simulink model "Final_Project"  (R2020b)
settings: Solver=VariableStepAuto  StartTime=0.0  StopTime=10.0  MaxStep=0.5e-5  RelTol=1e-3
libraries: nesl_utility x11, ee_lib x10, fl_lib x9, simulink x2
settings Model: Creator=edoardo  LastModifiedBy=edoardo
settings SolverCC: ZeroCrossAlgorithm=Adaptive
settings DebuggingCC: IgnoredZcDiagnostic=none

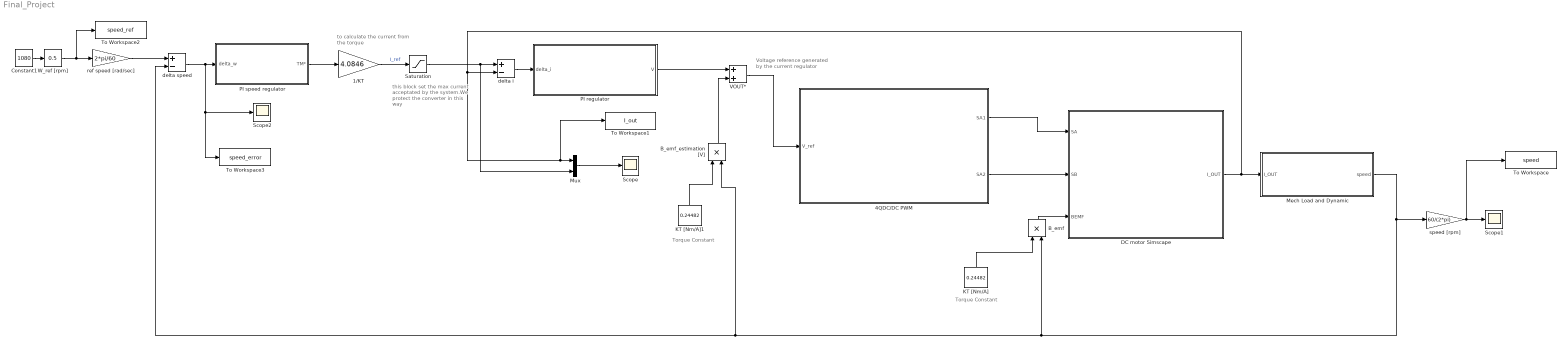
== system Final_Project ==
  note: Voltage reference generated
      | by the current regulator
  note: Torque Constant
  note: to calculate the current
      | from the torque
  note: this block set the max
      | current acceptated by the
      | system.We protect the
      | converter in this way
  note: Torque Constant
  " B_emf " : Product
  " B_emf_estimation [V]" : Product
  1/KT : Gain  Gain=4.0846
  4QDC/DC PWM : Subsystem
  Constant1 : Constant  Value=1080
  DC motor Simscape : Subsystem
  KT [Nm/A] : Constant  Value=0.24482
  KT [Nm/A]1 : Constant  Value=0.24482
  Mech Load and Dynamic : Subsystem
  Mux : Mux  Inputs=2
  PI regulator : Subsystem
  PI speed regulator : Subsystem
  Saturation : Saturate  UpperLimit=1.4  LowerLimit=-1.4
  Scope : Scope
  Scope1 : Scope
  Scope2 : Scope
  To Workspace : ToWorkspace  VariableName=speed  SaveFormat=Timeseries  SampleTime=-1
  To Workspace1 : ToWorkspace  VariableName=I_out  SaveFormat=Timeseries  SampleTime=-1
  To Workspace2 : ToWorkspace  VariableName=speed_ref  SaveFormat=Timeseries  SampleTime=-1
  To Workspace3 : ToWorkspace  VariableName=speed_error  SaveFormat=Timeseries  SampleTime=-1
  VOUT* : Sum
  W_ref [rpm] : simulink/Math Operations/Slider Gain  gain=0.5  low=-1  high=1
  "delta i " : Sum  Inputs=+-
  delta speed : Sum  Inputs=+-
  "ref speed [rad/sec] " : Gain  Gain=2*pi/60
  speed [rpm] : Gain  Gain=60/(2*pi)
  wires:
  KT [Nm/A]1/1 -> " B_emf_estimation [V]"/1
  " B_emf_estimation [V]"/1 -> VOUT*/2
  W_ref [rpm]/1 -> To Workspace2/1, "ref speed [rad/sec] "/1
  Constant1/1 -> W_ref [rpm]/1
  delta speed/1 -> Scope2/1, To Workspace3/1, PI speed regulator/1(delta_w)
  1/KT/1 -> Saturation/1  "I_ref"
  speed [rpm]/1 -> To Workspace/1, Scope1/1
  Saturation/1 -> Mux/2, "delta i "/1
  "ref speed [rad/sec] "/1 -> delta speed/1
  Mux/1 -> Scope/1
  DC motor Simscape/1(I_OUT) -> Mech Load and Dynamic/1(I_OUT), "delta i "/2, To Workspace1/1, Mux/1
  VOUT*/1 -> 4QDC/DC PWM/1(V_ref)
  "delta i "/1 -> PI regulator/1(delta_i)
  PI regulator/1(V) -> VOUT*/1
  PI speed regulator/1(TM*) -> 1/KT/1
  4QDC/DC PWM/1(SA1) -> DC motor Simscape/1(SA)
  4QDC/DC PWM/2(SA2) -> DC motor Simscape/2(SB)
  KT [Nm/A]/1 -> " B_emf "/1
  " B_emf "/1 -> DC motor Simscape/3(BEMF)
  Mech Load and Dynamic/1(speed) -> speed [rpm]/1, " B_emf "/2, " B_emf_estimation [V]"/2, delta speed/2

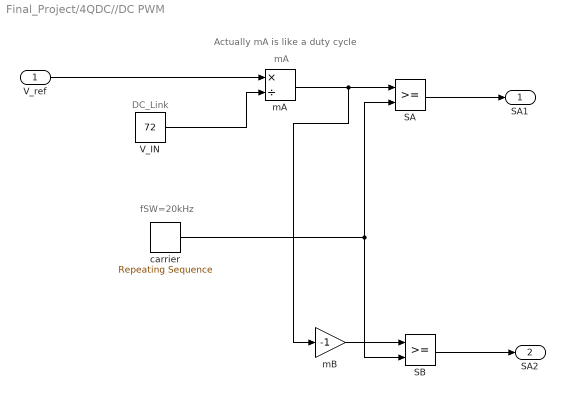
== system Final_Project/4QDC//DC PWM ==
  note: Actually mA is like a duty cycle
  note: DC_Link
  note: fSW=20kHz
  note: mA
  V_ref : Inport
  SA : RelationalOperator  OutDataTypeStr=boolean  RndMeth=Simplest
  SB : RelationalOperator  OutDataTypeStr=boolean  RndMeth=Simplest
  V_IN : Constant  Value=72
  carrier : simulink/Sources/Repeating Sequence  rep_seq_t=[0 0.5e-4/2 0.5e-4]  rep_seq_y=[-1 1 -1]
  mA : Product  Inputs=*/
  mB : Gain  Gain=-1
  SA1 : Outport
  SA2 : Outport  Port=2
  wires:
  V_ref/1 -> mA/1
  carrier/1 -> SA/2, SB/2
  mA/1 -> mB/1, SA/1
  SB/1 -> SA2/1
  mB/1 -> SB/1
  V_IN/1 -> mA/2
  SA/1 -> SA1/1

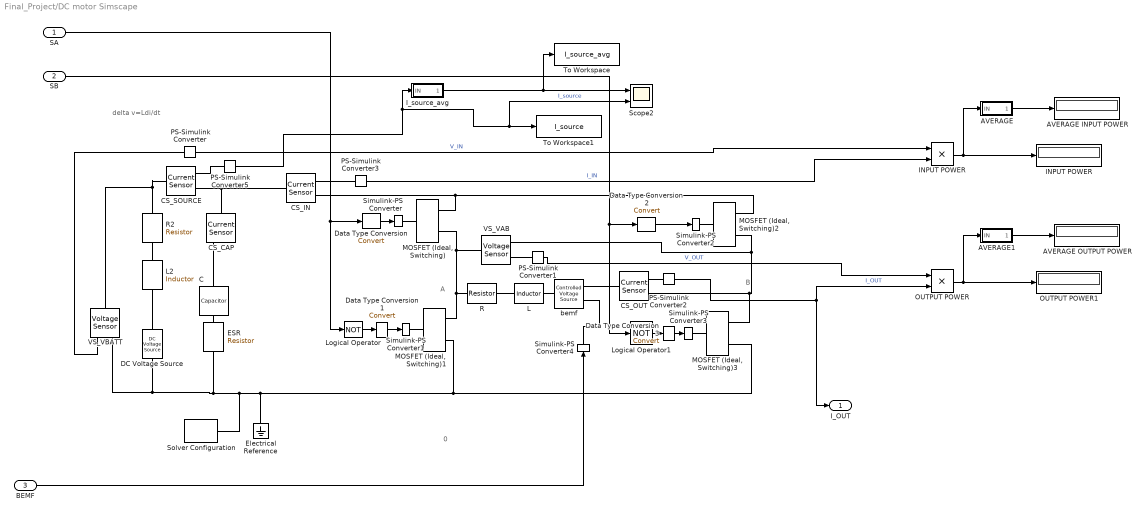
== system Final_Project/DC motor Simscape ==
  note: delta v=Ldi/dt
  note: B
  note: 0
  note: A
  SA : Inport
  SB : Inport  Port=2
  BEMF : Inport  Port=3
  " INPUT POWER" : Display
  AVERAGE : Subsystem  mask{Ts=0.0001}
      mask prompts: Ts "period"
  AVERAGE INPUT POWER : Display
  AVERAGE OUTPUT POWER : Display
  AVERAGE1 : Subsystem  mask{Ts=0.0001}
      mask prompts: Ts "period"
  C : ee_lib/Passive/Capacitor  cap_option=0  c=1e-4 F  Cvec=[1e-05, 1e-06] F  Vvec=[0, 10] V  CV_table_symmetry=1  f_vec=[1, 10] kHz  DFext_vec=[.8, 1.2]  C_tol=5  enable_C_tol=0  tol_distribution=1  nSigma=4  r=1e-6 Ohm  g=0 1/Ohm  averaging_period=0 s  enable_operating_limits=0  operating_limit_action=2  max_working_voltage_range=[-25, 25] V  power_rating=1 W  enable_faults=0  fault_action=1  Cscale_faulted=100  R_faulted=1e-3 Ohm  G_faulted=0 1/Ohm  tau_fault=1e-3 s  enable_temporal_fault=0  t_fault=1 s  enable_behavioral_fault=0  max_permissible_voltage_range=[-100, 100] V  t_fail_on_voltage=1 s  i_specify=off  i_priority=None  i=0 A  i_nominal_specify=off  i_nominal_unit=A  i_nominal_value=1  v_specify=off  v_priority=None  v=0 V  v_nominal_specify=off  v_nominal_unit=V  v_nominal_value=1  vc_specify=off  vc_priority=High  vc=0 V  vc_nominal_specify=off  vc_nominal_unit=V  vc_nominal_value=1
  CS_CAP : fl_lib/Electrical/Electrical Sensors/Current Sensor
  CS_IN : fl_lib/Electrical/Electrical Sensors/Current Sensor
  CS_OUT : fl_lib/Electrical/Electrical Sensors/Current Sensor
  CS_SOURCE : fl_lib/Electrical/Electrical Sensors/Current Sensor
  DC Voltage Source : fl_lib/Electrical/Electrical Sources/DC Voltage Source  v0=72 V
  Data Type Conversion{,1..3} (4 alike) : DataTypeConversion
  ESR : ee_lib/Passive/Resistor  R=0.01 Ohm  R_tol=5  enable_R_tol=0  tol_distribution=1  nSigma=4  enable_operating_limits=0  operating_limit_action=2  max_working_voltage=100 V  power_rating=1 W  enable_faults=0  fault_action=1  R_faulted=inf Ohm  enable_temporal_fault=0  t_fault=1 s  enable_behavioral_fault=0  max_permissible_current=1 A  t_fail_on_current=1 s  noise_mode=0  sample_time=1e-3 s  repeatability=1  auto_seed=3922919431  user_seed=0  Tdevice=25 degC  alpha=3.93e-3 1/K  Tmeas=25 degC  thermal_mass=100 J/K  power_derating_T1=70 degC  power_derating_T2=155 degC  operating_temperature_range_vec=[-50, 150] degC  temperature_specify=off  temperature_priority=High  temperature=298.15 K  temperature_nominal_specify=off  temperature_nominal_unit=K  temperature_nominal_value=1
  Electrical Reference : fl_lib/Electrical/Electrical Elements/Electrical Reference
  INPUT POWER : Product
  I_source_avg : Subsystem  mask{Ts=0.0001}
      mask prompts: Ts "period"
  L : ee_lib/Passive/Inductor  l=6.4e-3 H  L_tol=20  enable_L_tol=0  tol_distribution=1  nSigma=4  r=0 Ohm  g=1e-9 1/Ohm  enable_operating_limits=0  operating_limit_action=2  max_working_current=1 A  power_rating=1 W  enable_faults=0  fault_action=1  lambdaPercent=50  k_faulted=0.9999  turnsShort=0  openCct=0  groundShort=0  groundShortG=0 1/Ohm  tau_fault=1e-3 s  enable_temporal_fault=0  t_fault=1 s  enable_behavioral_fault=0  max_permissible_voltage=100 V  n_fail_on_voltage=1  max_permissible_current=1 A  t_fail_on_current=1 s  i_L_specify=off  i_L_priority=High  i_L=0 A  i_L_nominal_specify=off  i_L_nominal_unit=A  i_L_nominal_value=1
  L2 : ee_lib/Passive/Inductor  l=0.72e-3 H  L_tol=20  enable_L_tol=0  tol_distribution=1  nSigma=4  r=0 Ohm  g=1e-9 1/Ohm  enable_operating_limits=0  operating_limit_action=2  max_working_current=1 A  power_rating=1 W  enable_faults=0  fault_action=1  lambdaPercent=50  k_faulted=0.9999  turnsShort=0  openCct=0  groundShort=0  groundShortG=0 1/Ohm  tau_fault=1e-3 s  enable_temporal_fault=0  t_fault=1 s  enable_behavioral_fault=0  max_permissible_voltage=100 V  n_fail_on_voltage=1  max_permissible_current=1 A  t_fail_on_current=1 s  i_L_specify=off  i_L_priority=High  i_L=0 A  i_L_nominal_specify=off  i_L_nominal_unit=A  i_L_nominal_value=1
  Logical Operator : Logic  Operator=NOT  AllPortsSameDT=off  OutDataTypeStr=boolean
  Logical Operator1 : Logic  Operator=NOT  AllPortsSameDT=off  OutDataTypeStr=boolean
  MOSFET (Ideal, Switching){,1..3} (4 alike) : ee_lib/Semiconductors & Converters/MOSFET (Ideal, Switching)  Rds=0.1 Ohm  Goff=1e-6 1/Ohm  Vth=0.5 V  diode_param=1  diode_Vf=0.8 V  diode_Ron=0.001 Ohm  diode_Goff=1e-5 1/Ohm  diode_C=50e-9 F  diode_iRM=-235 A  diode_iF=300 A  diode_idot=-50 A/us  diode_trr_param=1  diode_trr_factor=3  diode_trr=15 us  diode_Qrr=1500 s*uA  thermal_loss_option=2  Von_data=[0, 1.1, 1.3, 1.45, 1.75, 2.25, 2.7; 0, 1, 1.15, 1.35, 1.7, 2.35, 3] V  Eon_data=[0, .29, 1.43, 2.86, 5.71, 13.14, 22.86; 0, .57, 2.63, 5.14, 10.29, 20.57, 30.29] * 1e-3 J  Eoff_data=[0, .21, 1.07, 2.14, 4.29, 9.86, 17.14; 0, .43, 1.97, 3.86, 7.71, 15.43, 22.71] * 1e-3 J  Tj=[298.15, 398.15] K  Iout_data=[0, 10, 50, 100, 200, 400, 600] A  Eon_scalar=22.86e-3 J  Eoff_scalar=17.14e-3 J  Voff=300 V  Iout_scalar=600 A  diodeModelType=ee.enum.converters.diodeModelType.pwl  diode_IfMat=[.07, .12, .19, 1.75, 4.24, 7.32, 11.2; .16, .3, .72, 2.14, 4.02, 6.35, 9.12] A  diode_TjVec=[25, 125] degC  diode_VfVec=[.5, .7, .9, 1.3, 1.7, 2.1, 2.5] V  thermal_network_parameterization=ee.enum.thermalNetworkTopology.external  Rth=[.03, .2] K/W  Rth_Foster=[.03, .2] K/W  thermal_mass_parameterization=ee.enum.thermalNetwork.timeconstant  thermal_mass=[3, 25] J/K  thermal_mass_Foster=[33, 50] J/K  thermal_time_constant=[.1, 5] s  thermal_time_constant_Foster=[1, 10] s  thermal_mass_initial_temperatures=[25, 25] degC  junction_thermal_mass=0.1 J/K  Tau=1e-4 s  vT_specify=off  vT_priority=None  vT=0 V  vT_nominal_specify=off  vT_nominal_unit=V  vT_nominal_value=1  Qj_specify=off  Qj_priority=None  Qj=0 W  Qj_nominal_specify=off  Qj_nominal_unit=W  Qj_nominal_value=1  junction_temperature_specify=off  junction_temperature_priority=None  junction_temperature=25 degC  junction_temperature_nominal_specify=off  junction_temperature_nominal_unit=degC  junction_temperature_nominal_value=1
  OUTPUT POWER : Product
  OUTPUT POWER1 : Display
  PS-Simulink Converter{,1..3,5} (5 alike) : nesl_utility/PS-Simulink Converter  PhysicalDomain=network_engine_domain  SubClassName=ps_output  LeftPortType=input  RightPortType=output  PseudoPeriodic=off  Frequencies=[]  Unit=1  AffineConversion=off
  R : ee_lib/Passive/Resistor  R=24.9 Ohm  R_tol=5  enable_R_tol=0  tol_distribution=1  nSigma=4  enable_operating_limits=0  operating_limit_action=2  max_working_voltage=100 V  power_rating=1 W  enable_faults=0  fault_action=1  R_faulted=inf Ohm  enable_temporal_fault=0  t_fault=1 s  enable_behavioral_fault=0  max_permissible_current=1 A  t_fail_on_current=1 s  noise_mode=0  sample_time=1e-3 s  repeatability=1  auto_seed=2715962282  user_seed=0  Tdevice=25 degC  alpha=3.93e-3 1/K  Tmeas=25 degC  thermal_mass=100 J/K  power_derating_T1=70 degC  power_derating_T2=155 degC  operating_temperature_range_vec=[-50, 150] degC  temperature_specify=off  temperature_priority=High  temperature=298.15 K  temperature_nominal_specify=off  temperature_nominal_unit=K  temperature_nominal_value=1
  R2 : ee_lib/Passive/Resistor  R=0.3 Ohm  R_tol=5  enable_R_tol=0  tol_distribution=1  nSigma=4  enable_operating_limits=0  operating_limit_action=2  max_working_voltage=100 V  power_rating=1 W  enable_faults=0  fault_action=1  R_faulted=inf Ohm  enable_temporal_fault=0  t_fault=1 s  enable_behavioral_fault=0  max_permissible_current=1 A  t_fail_on_current=1 s  noise_mode=0  sample_time=1e-3 s  repeatability=1  auto_seed=418932850  user_seed=0  Tdevice=25 degC  alpha=3.93e-3 1/K  Tmeas=25 degC  thermal_mass=100 J/K  power_derating_T1=70 degC  power_derating_T2=155 degC  operating_temperature_range_vec=[-50, 150] degC  temperature_specify=off  temperature_priority=High  temperature=298.15 K  temperature_nominal_specify=off  temperature_nominal_unit=K  temperature_nominal_value=1
  Scope2 : Scope  NumInputPorts=2
  Simulink-PS Converter{,1..4} (5 alike) : nesl_utility/Simulink-PS Converter  PhysicalDomain=network_engine_domain  SubClassName=ps_input  LeftPortType=input  RightPortType=output  PseudoPeriodic=off  Frequencies=[]  NoiseDistribution=none  NoiseParameters=[]  Unit=1  AffineConversion=off  FilteringAndDerivatives=provide  SimscapeFilterOrder=1  InputFilterTimeConstant=0.001  UdotUserProvided=0
  Solver Configuration : nesl_utility/Solver Configuration  PhysicalDomain=network_engine_domain  SubClassName=solver  LeftPortType=input  RightPortType=generic  Tones=[]  Harmonics=[]  SimulateNoise=off  Profile=off  UseLocalSampling=off  EnableSwitchedLinearOptims=on  FrequencyDomain=off  UseCCode=off  RelTol=0.001  AbsTol=1e-06  MinStep=1e-09  ToWorkspace=off  RevertToSquareIcSolve=off  NumHomotopyIterations=100  PhasorMode=off  PhasorModeNumHarmonics=1  DoDC=off  ResidualTolerance=1e-09  UseLocalSolver=off  LocalSolverChoice=NE_BACKWARD_EULER_ADVANCER  LocalSolverSampleTime=0.001  DoFixedCost=off  MaxNonlinIter=3  MaxModeIter=2  ComputeImpulses=off  ImpulseIterations=2  LinearAlgebra=auto  EquationFormulation=NE_TIME_EF  DelaysMemoryBudget=1024  AutomaticFiltering=on  FilteringTimeConstant=0.001  PartitionStorageMethod=AS_NEEDED  PartitionMemoryBudget=1024  PartitionMethod=ROBUST
  To Workspace : ToWorkspace  VariableName=I_source_avg  SaveFormat=Timeseries  SampleTime=-1
  To Workspace1 : ToWorkspace  VariableName=I_source  SaveFormat=Timeseries  SampleTime=-1
  VS_VAB : fl_lib/Electrical/Electrical Sensors/Voltage Sensor
  VS_VBATT : fl_lib/Electrical/Electrical Sensors/Voltage Sensor
  bemf : fl_lib/Electrical/Electrical Sources/Controlled Voltage Source
  I_OUT : Outport  VectorParamsAs1DForOutWhenUnconnected=off
  wires:
  BEMF/1 -> Simulink-PS Converter4/1
  PS-Simulink Converter2/1 -> I_OUT/1, OUTPUT POWER/2  "I_OUT"
  Data Type Conversion3/1 -> Simulink-PS Converter3/1
  PS-Simulink Converter3/1 -> INPUT POWER/2  "I_IN"
  Logical Operator/1 -> Data Type Conversion1/1
  SA/1 -> Logical Operator/1, Data Type Conversion/1
  SB/1 -> Data Type Conversion2/1, Logical Operator1/1
  Data Type Conversion/1 -> Simulink-PS Converter/1
  Data Type Conversion1/1 -> Simulink-PS Converter1/1
  PS-Simulink Converter/1 -> INPUT POWER/1  "V_IN"
  PS-Simulink Converter1/1 -> OUTPUT POWER/1  "V_OUT"
  Logical Operator1/1 -> Data Type Conversion3/1
  Data Type Conversion2/1 -> Simulink-PS Converter2/1
  PS-Simulink Converter5/1 -> I_source_avg/1(IN), Scope2/2, To Workspace1/1  "I_source"
  I_source_avg/1(OUT) -> To Workspace/1, Scope2/1
  INPUT POWER/1 -> AVERAGE/1(IN), " INPUT POWER"/1
  AVERAGE/1(OUT) -> AVERAGE INPUT POWER/1
  OUTPUT POWER/1 -> AVERAGE1/1(IN), OUTPUT POWER1/1
  AVERAGE1/1(OUT) -> AVERAGE OUTPUT POWER/1
  connections:
  Simulink-PS Converter1/RConn1 -- "MOSFET (Ideal, Switching)1"/LConn1
  CS_IN/LConn1 -- CS_SOURCE/RConn2 -- CS_CAP/LConn1
  CS_IN/RConn1 -- PS-Simulink Converter3/LConn1
  "MOSFET (Ideal, Switching)"/RConn2 -- R/LConn1 -- "MOSFET (Ideal, Switching)1"/RConn1 -- VS_VAB/LConn1
  CS_OUT/RConn1 -- PS-Simulink Converter2/LConn1
  bemf/LConn1 -- L/RConn1
  VS_VBATT/RConn1 -- PS-Simulink Converter/LConn1
  Simulink-PS Converter2/RConn1 -- "MOSFET (Ideal, Switching)2"/LConn1
  "MOSFET (Ideal, Switching)2"/RConn2 -- VS_VAB/RConn2 -- CS_OUT/RConn2 -- "MOSFET (Ideal, Switching)3"/RConn1
  bemf/RConn2 -- CS_OUT/LConn1
  CS_IN/RConn2 -- "MOSFET (Ideal, Switching)2"/RConn1 -- "MOSFET (Ideal, Switching)"/RConn1
  L/LConn1 -- R/RConn1
  Simulink-PS Converter4/RConn1 -- bemf/RConn1
  Simulink-PS Converter/RConn1 -- "MOSFET (Ideal, Switching)"/LConn1
  PS-Simulink Converter1/LConn1 -- VS_VAB/RConn1
  Simulink-PS Converter3/RConn1 -- "MOSFET (Ideal, Switching)3"/LConn1
  DC Voltage Source/LConn1 -- L2/RConn1
  L2/LConn1 -- R2/RConn1
  C/RConn1 -- ESR/LConn1
  CS_CAP/RConn2 -- C/LConn1
  R2/LConn1 -- CS_SOURCE/LConn1 -- VS_VBATT/LConn1
  PS-Simulink Converter5/LConn1 -- CS_SOURCE/RConn1
  "MOSFET (Ideal, Switching)3"/RConn2 -- "MOSFET (Ideal, Switching)1"/RConn2 -- Electrical Reference/LConn1 -- VS_VBATT/RConn2 -- DC Voltage Source/RConn1 -- ESR/RConn1 -- Solver Configuration/RConn1

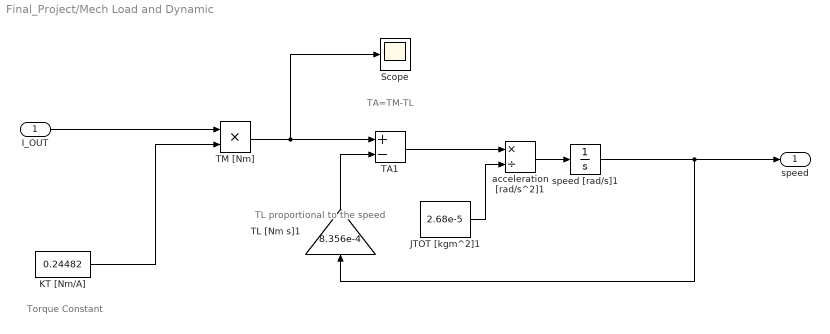
== system Final_Project/Mech Load and Dynamic ==
  note: TL proportional
      | to the speed
  note: TA=TM-TL
  note: Torque Constant
  I_OUT : Inport
  JTOT [kgm^2]1 : Constant  Value=2.68e-5
  KT [Nm/A] : Constant  Value=0.24482
  Scope : Scope
  TA1 : Sum  Inputs=+-
  TL [Nm s]1 : Gain  Gain=8.356e-4
  TM [Nm] : Product
  acceleration [rad/s^2]1 : Product  Inputs=*/
  speed [rad/s]1 : Integrator
  speed : Outport
  wires:
  speed [rad/s]1/1 -> TL [Nm s]1/1, speed/1
  TA1/1 -> acceleration [rad/s^2]1/1
  acceleration [rad/s^2]1/1 -> speed [rad/s]1/1
  JTOT [kgm^2]1/1 -> acceleration [rad/s^2]1/2
  TL [Nm s]1/1 -> TA1/2
  I_OUT/1 -> TM [Nm]/1
  TM [Nm]/1 -> Scope/1, TA1/1
  KT [Nm/A]/1 -> TM [Nm]/2

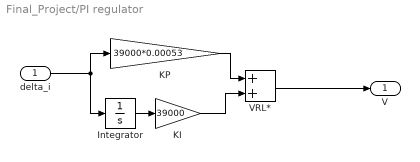
== system Final_Project/PI regulator ==
  delta_i : Inport
  Integrator : Integrator
  KI : Gain  Gain=39000
  KP : Gain  Gain=39000*0.00053
  VRL* : Sum
  V : Outport
  wires:
  Integrator/1 -> KI/1
  KI/1 -> VRL*/2
  VRL*/1 -> V/1
  delta_i/1 -> Integrator/1, KP/1
  KP/1 -> VRL*/1

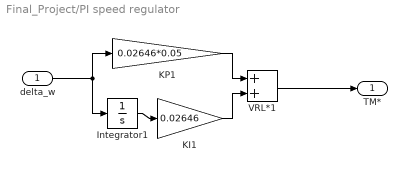
== system Final_Project/PI speed regulator ==
  delta_w : Inport
  Integrator1 : Integrator
  KI1 : Gain  Gain=0.02646
  KP1 : Gain  Gain=0.02646*0.05
  VRL*1 : Sum
  TM* : Outport
  wires:
  Integrator1/1 -> KI1/1
  VRL*1/1 -> TM*/1
  delta_w/1 -> Integrator1/1, KP1/1
  KI1/1 -> VRL*1/2
  KP1/1 -> VRL*1/1

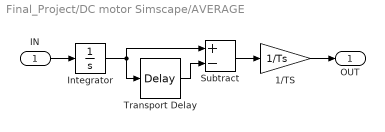
== system Final_Project/DC motor Simscape/AVERAGE ==
  IN : Inport
  1/TS : Gain  Gain=1/Ts
  Integrator : Integrator
  Subtract : Sum  Inputs=+-
  Transport Delay : TransportDelay  DelayTime=Ts
  OUT : Outport  VectorParamsAs1DForOutWhenUnconnected=off
  wires:
  Subtract/1 -> 1/TS/1
  Transport Delay/1 -> Subtract/2
  IN/1 -> Integrator/1
  1/TS/1 -> OUT/1
  Integrator/1 -> Subtract/1, Transport Delay/1

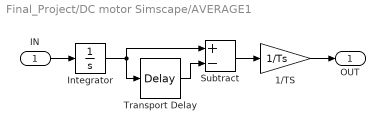
== system Final_Project/DC motor Simscape/AVERAGE1 ==
  IN : Inport
  1/TS : Gain  Gain=1/Ts
  Integrator : Integrator
  Subtract : Sum  Inputs=+-
  Transport Delay : TransportDelay  DelayTime=Ts
  OUT : Outport  VectorParamsAs1DForOutWhenUnconnected=off
  wires:
  Subtract/1 -> 1/TS/1
  Transport Delay/1 -> Subtract/2
  IN/1 -> Integrator/1
  1/TS/1 -> OUT/1
  Integrator/1 -> Subtract/1, Transport Delay/1

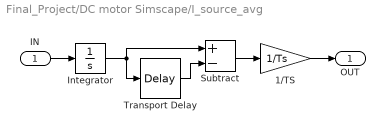
== system Final_Project/DC motor Simscape/I_source_avg ==
  IN : Inport
  1/TS : Gain  Gain=1/Ts
  Integrator : Integrator
  Subtract : Sum  Inputs=+-
  Transport Delay : TransportDelay  DelayTime=Ts
  OUT : Outport  VectorParamsAs1DForOutWhenUnconnected=off
  wires:
  Subtract/1 -> 1/TS/1
  Transport Delay/1 -> Subtract/2
  IN/1 -> Integrator/1
  1/TS/1 -> OUT/1
  Integrator/1 -> Subtract/1, Transport Delay/1
